simulink model "LabFD_CLFreqResponse"  (R2016a)
settings: Solver=VariableStepAuto  StartTime=0.0  StopTime=20  RelTol=1e-3
settings Model: Creator=jordan  LastModifiedBy=jordan

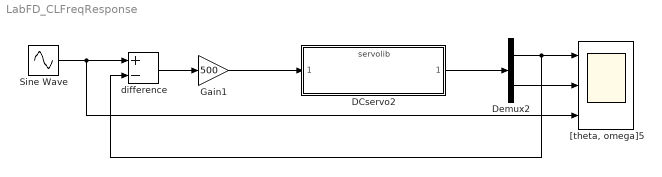
== system LabFD_CLFreqResponse ==
  DCservo2 : ModelReference  ModelNameDialog=servolib.slx  SimulationMode=Normal  ModelReferenceVersion=1.70
  Demux2 : Demux  Outputs=2
  Gain1 : Gain  Gain=500
  Sine Wave : Sin  Frequency=15  SampleTime=0
  "[theta, omega]5" : Scope  NumInputPorts=3
  difference : Sum  Inputs=+-
  wires:
  DCservo2/1 -> Demux2/1
  Demux2/2 -> "[theta, omega]5"/2
  Demux2/1 -> difference/2, "[theta, omega]5"/1
  Gain1/1 -> DCservo2/1
  difference/1 -> Gain1/1
  Sine Wave/1 -> "[theta, omega]5"/3, difference/1
